simulink model "decoupling_hamna_final"  (R2025b)
settings: Solver=VariableStepAuto  StartTime=0.0  StopTime=10.0  RelTol=1e-3
settings Model: Creator=3 Stars Laptop  LastModifiedBy=3 Stars Laptop

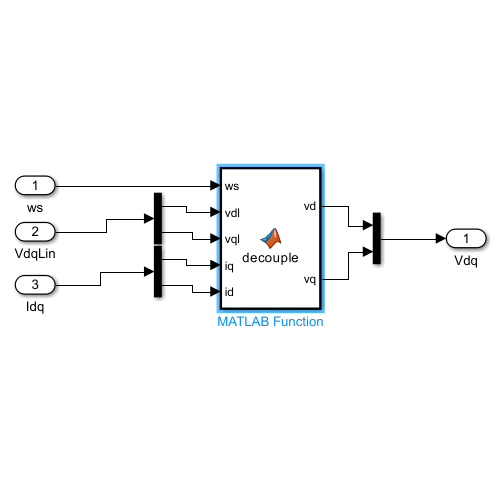
[thumbnail: Simulink's stored preview of the top-level diagram]
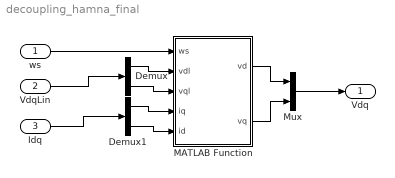
== system decoupling_hamna_final ==
  ws : Inport
  VdqLin : Inport  Port=2
  Idq : Inport  Port=3
  Demux : Demux  Outputs=2
  Demux1 : Demux  Outputs=2
  MATLAB Function : MATLAB Function  TreatAsAtomicUnit=on
  Mux : Mux  Inputs=2
  Vdq : Outport
  wires:
  ws/1 -> MATLAB Function/1(ws)
  VdqLin/1 -> Demux/1
  Demux/1 -> MATLAB Function/2(vdl)
  Demux/2 -> MATLAB Function/3(vql)
  Idq/1 -> Demux1/1
  Demux1/1 -> MATLAB Function/4(iq)
  Demux1/2 -> MATLAB Function/5(id)
  MATLAB Function/1(vd) -> Mux/1
  MATLAB Function/2(vq) -> Mux/2
  Mux/1 -> Vdq/1

== matlab function decoupling_hamna_final/MATLAB Function ==
  data: ws input; vd output; vdl input; vql input; iq input; id input; vq output
function [vd,vq]= decouple(ws,vdl,vql,iq,id)
Ld = 1e-4;
Lq = 1e-3;
phi = 0.23;
vd = -ws*Lq*iq + vdl*Ld;
vq = ws*phi + ws*Ld*id + vql*Lq;
